simulink model "sf_fxptprecision"  (Simulink 6.0)
settings: Solver=FixedStepDiscrete  StartTime=0.0  StopTime=1  FixedStep=1  RelTol=1e-3
settings Model: CovMetricSettings=dcmtr  Creator=The MathWorks Inc.  LastModifiedBy=batserve  ExtModeAutoUpdateStatusClock=off
settings DebuggingCC: CheckExecutionContextPreStartOutputMsg=on  CheckExecutionContextRuntimeOutputMsg=on  SolverPrmCheckMsg=none
settings HardwareCC: TargetUnknown=on

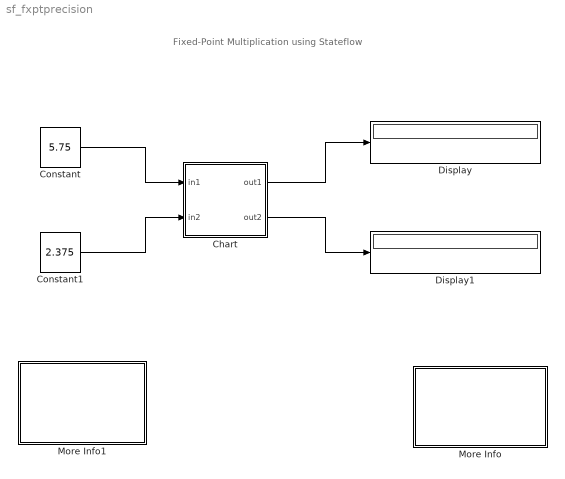
== system sf_fxptprecision ==
  note: Fixed-Point Multiplication using Stateflow
  Chart : Stateflow chart  PropExecContextAcrossSSBoundary=on
  Constant : Constant  Value=5.75  OutDataTypeMode=Specify via dialog  OutDataType=ufix(8)  OutScaling=2^-2
  Constant1 : Constant  Value=2.375  OutDataTypeMode=Specify via dialog  OutDataType=ufix(8)  OutScaling=2^-3
  Display : Display
  Display1 : Display
  More Info : Subsystem  PropExecContextAcrossSSBoundary=on
      mask Display: disp('Double click\nhere for\ninformation on\nthis demonstration')
  More Info1 : Subsystem  PropExecContextAcrossSSBoundary=on
      settings: OpenFcn=simcad(bdroot);
      mask Display: disp('Double click\nhere for\nSimulink\Stateflow\n Help')
  wires:
  Constant/1 -> Chart/1(in1)
  Constant1/1 -> Chart/2(in2)
  Chart/1(out1) -> Display/1
  Chart/2(out2) -> Display1/1

== system sf_fxptprecision/More Info ==
  note: Fixed-Point Multiplication
  note: This demonstration illustrates how Fixed-Point mathematics can be used within
      | your Stateflow chart. The chart takes two fixed-point inputs from Simulink: 'in1' is an
      | unsigned 8 bit integer with a slope bias of 2^-2 and 'in2' is an unsigned 8 bit integer
      | with a slope bias of 2^-3. The chart provides two outputs: 'out1' which is an unsigned
      | 8 bit integer with a slope bias of 2^-2 and 'out2' which is an unsigned 8 bit integer with
      | a slope bias of 2^-4.
      |
      | 'out1' and 'out2' are calculated the same way: in1 * in2. This model demonstrates how you
      | obtain different results when specifiying different values for your fixed-point output. In this
      | particular case, 'out2' is more accurate than 'out1' but is still a truncated result. In order to
      | obtain the correct result, you need to increase the bit (or register) size of the output and also
      | increase the slope bias (in other words shift the radix point). For example, if you select the
      | Data properties of 'out2' and change the integer size to a uint16 with a scaling value of 2^-5,
      | then you will receive the correct result:   13.65625

== system sf_fxptprecision/More Info1 ==

== stateflow chart Chart ==
  (default) -> (junction 3) : {out1=in1*in2;}
  (junction 3) -> (junction 4) : {out2=in1*in2;}
  data: in1 input fixpt; in2 input fixpt; out1 output fixpt; out2 output fixpt
